simulink library "calcNormalizedPathCoord_ul"  (R2020a)
settings: Solver=VariableStepAuto  StartTime=0.0  StopTime=10.0  RelTol=1e-3
settings Model: Creator=Ayaz  LastModifiedBy=Ayaz

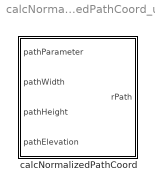
== system calcNormalizedPathCoord_ul ==
  calcNormalizedPathCoord : Subsystem

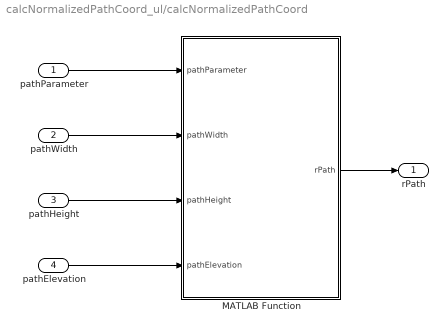
== system calcNormalizedPathCoord_ul/calcNormalizedPathCoord ==
  pathParameter : Inport
  pathWidth : Inport  Port=2
  pathHeight : Inport  Port=3
  pathElevation : Inport  Port=4
  MATLAB Function : MATLAB Function  TreatAsAtomicUnit=on
  rPath : Outport
  wires:
  pathElevation/1 -> MATLAB Function/4(pathElevation)
  pathHeight/1 -> MATLAB Function/3(pathHeight)
  pathWidth/1 -> MATLAB Function/2(pathWidth)
  pathParameter/1 -> MATLAB Function/1(pathParameter)
  MATLAB Function/1(rPath) -> rPath/1

== matlab function calcNormalizedPathCoord_ul/calcNormalizedPathCoord/MATLAB Function ==
  data: pathParameter input; rPath output; pathWidth input; pathHeight input; pathElevation input
function rPath = calcNormalizedPathCoords(pathParameter,...
    pathWidth,pathHeight,pathElevation)

rPath = calcNormalizedPathCoords(pathParameter,...
    pathWidth,pathHeight,pathElevation);

end
